simulink model "Ackermann_kinematic_model"  (R2024b)
settings: Solver=FixedStepAuto  StartTime=0.0  StopTime=10.0  FixedStep=1e-5  RelTol=1e-3
values from neighbouring files (symbols this model uses):
  L = 250e-3    (= 0.25)    [Init_parameters_kinematic.m]
  phi = [0,0.1]    [Init_parameters_kinematic.m]
  theta = 0    [Init_parameters_kinematic.m]
  x = 0    [Init_parameters_kinematic.m]
  y = 0    [Init_parameters_kinematic.m]
settings Model: Creator=Nabil  LastModifiedBy=Nabil

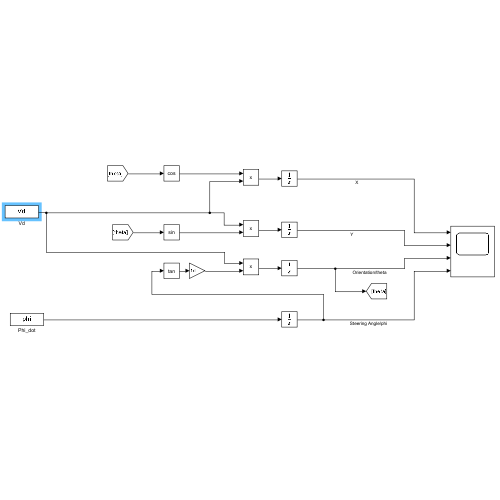
[thumbnail: Simulink's stored preview of the top-level diagram]
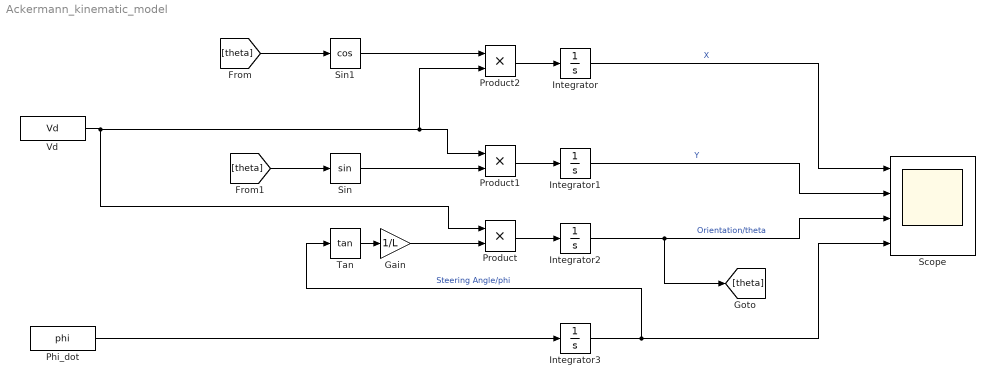
== system Ackermann_kinematic_model ==
  Gain : Gain  Gain=1/L
  Integrator : Integrator  InitialCondition=x
  Integrator1 : Integrator  InitialCondition=y
  Integrator2 : Integrator  InitialCondition=theta
  Integrator3 : Integrator  InitialCondition=phi
  Phi_dot : FromWorkspace  VariableName=phi
  Product : Product
  Product1 : Product
  Product2 : Product
  Scope : Scope  NumInputPorts=4
  Sin : Trigonometry
  Sin1 : Trigonometry  Operator=cos
  Tan : Trigonometry  Operator=tan
  Vd : FromWorkspace  VariableName=Vd
  wires:
  Integrator/1 -> Scope/1  "X"
  Integrator1/1 -> Scope/2  "Y"
  Integrator2/1 -> [theta], Scope/3  "Orientation/theta"
  Integrator3/1 -> Tan/1, Scope/4  "Steering Angle/phi"
  Phi_dot/1 -> Integrator3/1
  Tan/1 -> Gain/1
  Product/1 -> Integrator2/1
  Gain/1 -> Product/2
  Product1/1 -> Integrator1/1
  Product2/1 -> Integrator/1
  Sin/1 -> Product1/2
  Vd/1 -> Product/1, Product2/2, Product1/1
  Sin1/1 -> Product2/1
  [theta] -> Sin1/1
  [theta] -> Sin/1
